simulink model "mod_win_validation"  (R2023b)
settings: Solver=FixedStepAuto  StartTime=0.0  StopTime=10  FixedStep=0.001  RelTol=1e-3
values from neighbouring files (symbols this model uses):
  atan_scale = 100    [threeDiskOscillator.m]    (also in timing_calc.m)
  b_1 = mean(ECP_values([6 7]))    [threeDiskOscillator.m]    (also in timing_calc.m)
  b_2 = mean(ECP_values([8 9]))    [threeDiskOscillator.m]    (also in timing_calc.m)
  b_3 = mean(ECP_values([10 11]))    [threeDiskOscillator.m]    (also in timing_calc.m)
  C = [  1 0 0 0 0 0 ... (first row only)    [threeDiskOscillator.m]    (also in timing_calc.m = [)
  C_kf_aug = [C zeros(3,1)]    [timing_calc.m]
  C_ref = []    [threeDiskOscillator.m]    (also in timing_calc.m = pinv(C_3*inv(eye(6) - F + G*K_discr)*G*K_discr))
  F_kf_aug = [F_d G_d(:,1);zeros(1,6) 1]    [timing_calc.m]
  G_kf_aug = [G_d;0 0]    [timing_calc.m]
  J_1 = ECP_values(1)    [threeDiskOscillator.m]    (also in timing_calc.m)
  J_2 = ECP_values(2)    [threeDiskOscillator.m]    (also in timing_calc.m)
  J_3 = ECP_values(3)    [threeDiskOscillator.m]    (also in timing_calc.m)
  k_1 = ECP_values(4)    [threeDiskOscillator.m]    (also in timing_calc.m)
  k_2 = ECP_values(5)    [threeDiskOscillator.m]    (also in timing_calc.m)
  L_kf_aug = dlqe(F_kf_aug,eye(7),C_kf_aug,1e-3*eye(7),                  sigma_meas(1,1).^2*eye(3))    [timing_calc.m]
  sigma_meas = 0.0093*eye(3)    [threeDiskOscillator.m]    (also in timing_calc.m)
  T_Cm = ECP_values(13)    [threeDiskOscillator.m]    (also in timing_calc.m)
  T_Cp = ECP_values(12)    [threeDiskOscillator.m]    (also in timing_calc.m)
  T_s = 0.004    [threeDiskOscillator.m]    (also in timing_calc.m)
  w_th = 0.75    [threeDiskOscillator.m]    (also in timing_calc.m)
  x_0 = [0;0;0;0;0;0]    [threeDiskOscillator.m]    (also in timing_calc.m)
undefined symbols (not defined in the file or in its folder): K_discr, Serial_Port, Standard_Devices
libraries: sldrtlib x3, simulink x1
settings Model: Creator=farfar  LastModifiedBy=farfar
settings DataIOCC: SaveFormat=Array  ReturnWorkspaceOutputs=off  TimeSaveName=t
settings HardwareCC: ProdBitPerLong=64  ProdHWDeviceType=Intel->x86-64 (Linux 64)
settings RTWCC: Description=Simulink Desktop Real-Time  SystemTargetFile=sldrt.tlc  TemplateMakefile=sldrt.tmf  RTWCompilerOptimization=on
settings CodeAppCC: MaxIdLength=95
settings SimulinkDesktopRealTimeCC: TargetLibSuffix=_sldrt.a  TargetPreCompLibLocation=C:\Program Files\MATLAB\R2023b\toolbox\sldrt\lib\win64

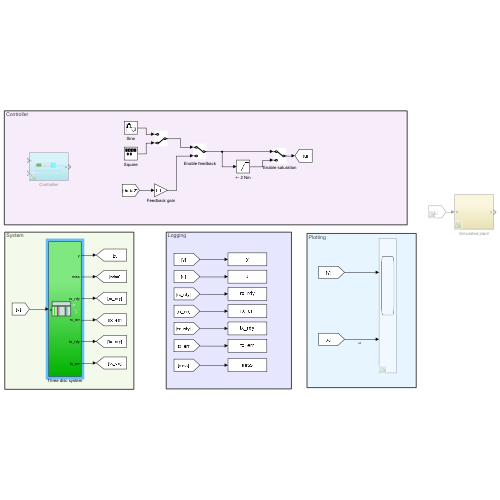
[thumbnail: Simulink's stored preview of the top-level diagram]
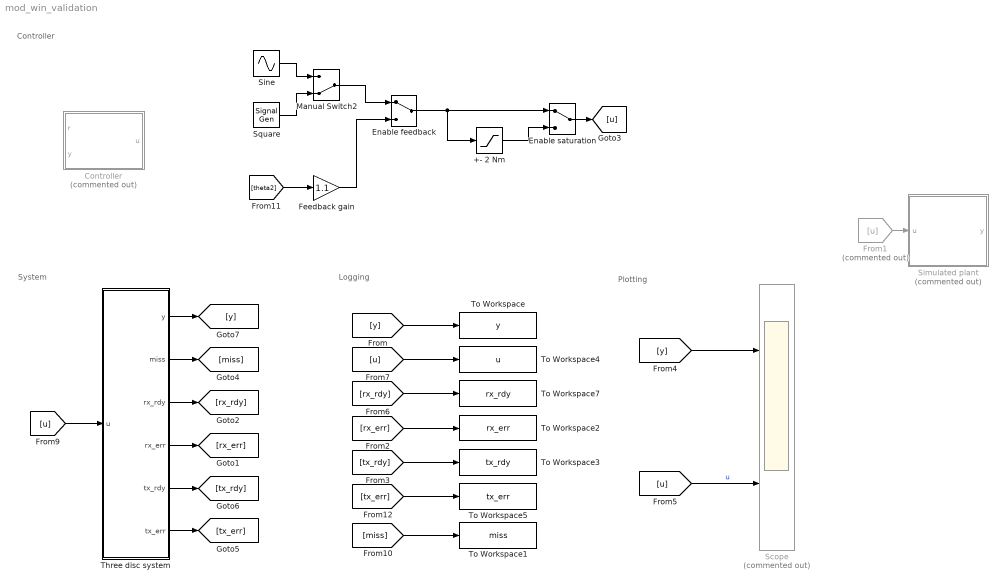
== system mod_win_validation ==
  note: Controller
  note: Plotting
  note: System
  note: Logging
  +- 2 Nm : Saturate  UpperLimit=2.0  LowerLimit=-2.0
  Controller : Subsystem  Commented=on
  Enable feedback : ManualSwitch
  Enable saturation : ManualSwitch
  Feedback gain : Gain  Gain=1.1
  From1 : From  Commented=on  GotoTag=u
  Manual Switch2 : ManualSwitch  CurrentSetting=0
  Scope : Scope  Commented=on  NumInputPorts=2
  Simulated plant : Subsystem  Commented=on
  Sine : Sin  Amplitude=0.1  Frequency=0.25*2*pi  SampleTime=0.004
  Square : SignalGenerator  WaveForm=square  Amplitude=0.1  Frequency=1/(20*0.004)
  Three disc system : Subsystem
  To Workspace : ToWorkspace  VariableName=y  SampleTime=0.001
  To Workspace1 : ToWorkspace  VariableName=miss  SampleTime=0.001
  To Workspace2 : ToWorkspace  VariableName=rx_err  SampleTime=0.001
  To Workspace3 : ToWorkspace  VariableName=tx_rdy  SampleTime=0.001
  To Workspace4 : ToWorkspace  VariableName=u  SampleTime=0.001
  To Workspace5 : ToWorkspace  VariableName=tx_err  SampleTime=0.001
  To Workspace7 : ToWorkspace  VariableName=rx_rdy  SampleTime=0.001
  wires:
  Three disc system/2(miss) -> [miss]
  Three disc system/1(y) -> [y]
  [y] -> To Workspace/1
  [u] -> To Workspace4/1
  [miss] -> To Workspace1/1
  From1/1 -> Simulated plant/1(u)
  Three disc system/3(rx_rdy) -> [rx_rdy]
  Three disc system/4(rx_err) -> [rx_err]
  [u] -> Three disc system/1(u)
  Enable feedback/1 -> Enable saturation/1, +- 2 Nm/1
  +- 2 Nm/1 -> Enable saturation/2
  Enable saturation/1 -> [u]
  [rx_rdy] -> To Workspace7/1
  Manual Switch2/1 -> Enable feedback/1
  Sine/1 -> Manual Switch2/1
  Square/1 -> Manual Switch2/2
  [theta2] -> Feedback gain/1
  Feedback gain/1 -> Enable feedback/2
  [u] -> Scope/2  "u"
  [y] -> Scope/1
  Three disc system/6(tx_err) -> [tx_err]
  Three disc system/5(tx_rdy) -> [tx_rdy]
  [rx_err] -> To Workspace2/1
  [tx_rdy] -> To Workspace3/1
  [tx_err] -> To Workspace5/1

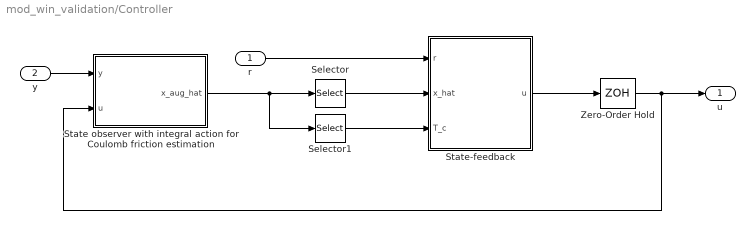
== system mod_win_validation/Controller ==
  r : Inport
  y : Inport  Port=2
  Selector : Selector  InputPortWidth=7  IndexOptions=Index vector (dialog)  Indices=[1:6]  OutputSizes=1
  Selector1 : Selector  InputPortWidth=7  IndexOptions=Index vector (dialog)  Indices=[7]  OutputSizes=1
  State observer with integral action for Coulomb friction estimation : Subsystem
  State-feedback : Subsystem
  Zero-Order Hold : ZeroOrderHold  SampleTime=T_s
  u : Outport
  wires:
  r/1 -> State-feedback/1(r)
  Zero-Order Hold/1 -> State observer with integral action for Coulomb friction estimation/2(u), u/1
  Selector1/1 -> State-feedback/3(T_c)
  Selector/1 -> State-feedback/2(x_hat)
  State-feedback/1(u) -> Zero-Order Hold/1
  y/1 -> State observer with integral action for Coulomb friction estimation/1(y)
  State observer with integral action for Coulomb friction estimation/1(x_aug_hat) -> Selector1/1, Selector/1

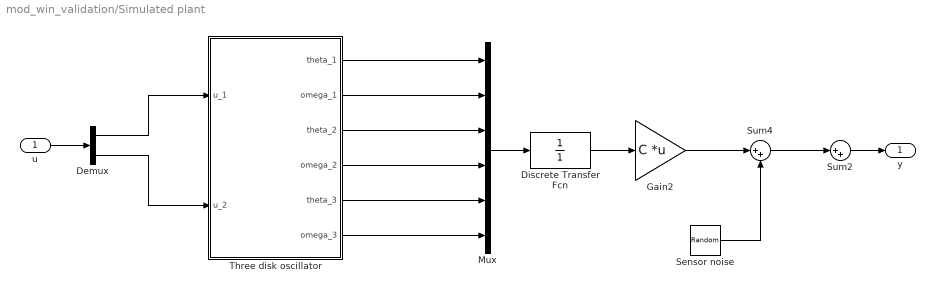
== system mod_win_validation/Simulated plant ==
  u : Inport
  Demux : Demux  Outputs=2
  Discrete Transfer Fcn : DiscreteTransferFcn  Denominator=[1]  SampleTime=T_s
  Gain2 : Gain  Gain=C  Multiplication=Matrix(K*u) (u vector)
  Mux : Mux  Inputs=6
  Sensor noise : RandomNumber  Mean=zeros(3,1)  Variance=diag(sigma_meas^2)  SampleTime=T_s
  Sum2 : Sum  Inputs=|++
  Sum4 : Sum  Inputs=|++
  Three disk oscillator : Subsystem
  y : Outport  VectorParamsAs1DForOutWhenUnconnected=off
  wires:
  u/1 -> Demux/1
  Three disk oscillator/2(omega_1) -> Mux/2
  Three disk oscillator/1(theta_1) -> Mux/1
  Mux/1 -> Discrete Transfer Fcn/1
  Three disk oscillator/4(omega_2) -> Mux/4
  Three disk oscillator/3(theta_2) -> Mux/3
  Discrete Transfer Fcn/1 -> Gain2/1
  Gain2/1 -> Sum4/1
  Sum4/1 -> Sum2/1
  Sensor noise/1 -> Sum4/2
  Three disk oscillator/6(omega_3) -> Mux/6
  Three disk oscillator/5(theta_3) -> Mux/5
  Sum2/1 -> y/1
  Demux/1 -> Three disk oscillator/1(u_1)
  Demux/2 -> Three disk oscillator/2(u_2)

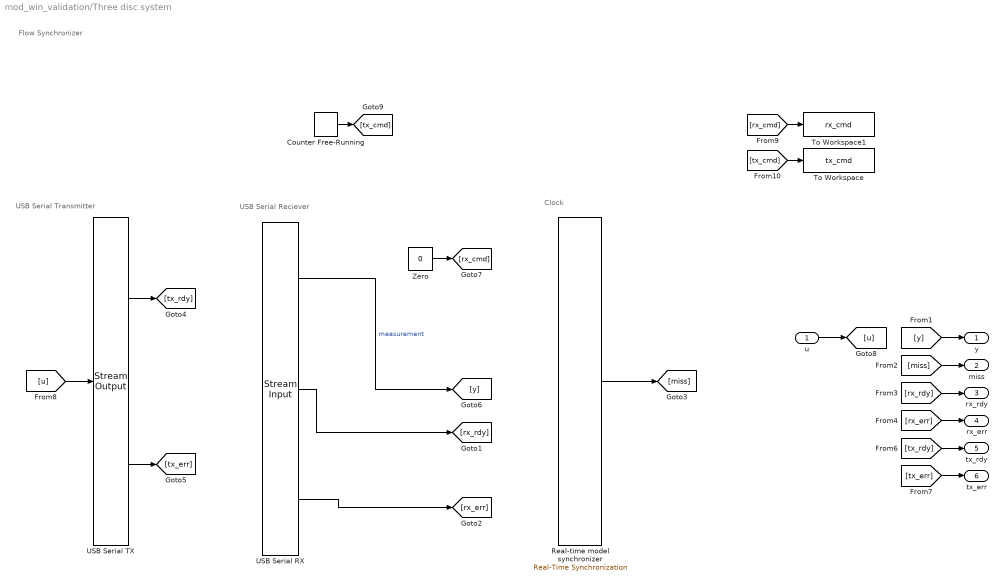
== system mod_win_validation/Three disc system ==
  note: Flow Synchronizer
  note: USB Serial Transmitter
  note: USB Serial Reciever
  note: Clock
  u : Inport
  Counter Free-Running : simulink/Sources/Counter Free-Running  NumBits=32  tsamp=0.004
  Real-time model synchronizer : sldrtlib/Real-Time Synchronization  SampleTime=0.001  MaxMissedTicks=10000  ShowMissedTicks=on  YieldWhenWaiting=off
  To Workspace : ToWorkspace  VariableName=tx_cmd  SampleTime=0.001
  To Workspace1 : ToWorkspace  VariableName=rx_cmd  SampleTime=0.001
  USB Serial RX : sldrtlib/Stream Input  SampleTime=0.001  MaxMissedTicks=10000  ShowMissedTicks=off  YieldWhenWaiting=off  DrvName=Standard_Devices/Serial_Port  DrvAddress=8  DrvOptions=[12000000 8 0 0 0 0 0 0]  DataTypes={'3*double'}  FormatString='%f %f %f'  Terminator={'\n'}  ShowReady=on  ShowError=on
      settings: AttributesFormatString=Serial Port [8]
  USB Serial TX : sldrtlib/Stream Output  SampleTime=0.004  MaxMissedTicks=1000  ShowMissedTicks=off  YieldWhenWaiting=off  DrvName=Standard_Devices/Serial_Port  DrvAddress=8  DrvOptions=[12000000 8 0 0 0 0 0 0]  PortSizes=[1]  FormatString='%f\n'  ShowReady=on  ShowError=on  InitialValue='B\n'  FinalValue='S\n'
      settings: AttributesFormatString=Serial Port [8]
  Zero : Constant  Value=0  OutDataTypeStr=Inherit: Inherit via back propagation
  y : Outport
  miss : Outport  Port=2
  rx_rdy : Outport  Port=3
  rx_err : Outport  Port=4
  tx_rdy : Outport  Port=5
  tx_err : Outport  Port=6
  wires:
  USB Serial TX/1 -> [tx_rdy]
  USB Serial RX/1 -> [y]  "measurement"
  [y] -> y/1
  u/1 -> [u]
  USB Serial RX/3 -> [rx_err]
  Real-time model synchronizer/1 -> [miss]
  [miss] -> miss/1
  [rx_rdy] -> rx_rdy/1
  [rx_err] -> rx_err/1
  USB Serial TX/2 -> [tx_err]
  [tx_err] -> tx_err/1
  [tx_rdy] -> tx_rdy/1
  [u] -> USB Serial TX/1
  Counter Free-Running/1 -> [tx_cmd]
  [rx_cmd] -> To Workspace1/1
  [tx_cmd] -> To Workspace/1
  Zero/1 -> [rx_cmd]
  USB Serial RX/2 -> [rx_rdy]

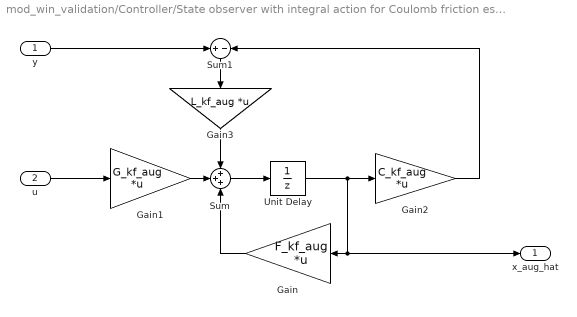
== system mod_win_validation/Controller/State observer with integral action for Coulomb friction estimation ==
  y : Inport
  u : Inport  Port=2
  Gain : Gain  Gain=F_kf_aug  Multiplication=Matrix(K*u) (u vector)
  Gain1 : Gain  Gain=G_kf_aug  Multiplication=Matrix(K*u) (u vector)
  Gain2 : Gain  Gain=C_kf_aug  Multiplication=Matrix(K*u) (u vector)
  Gain3 : Gain  Gain=L_kf_aug  Multiplication=Matrix(K*u) (u vector)
  Sum : Sum  Inputs=+++
  Sum1 : Sum  Inputs=+-
  Unit Delay : UnitDelay  SampleTime=T_s  HasFrameUpgradeWarning=on
  x_aug_hat : Outport  VectorParamsAs1DForOutWhenUnconnected=off
  wires:
  Unit Delay/1 -> x_aug_hat/1, Gain/1, Gain2/1
  y/1 -> Sum1/1
  Sum1/1 -> Gain3/1
  Sum/1 -> Unit Delay/1
  Gain2/1 -> Sum1/2
  u/1 -> Gain1/1
  Gain1/1 -> Sum/2
  Gain/1 -> Sum/3
  Gain3/1 -> Sum/1

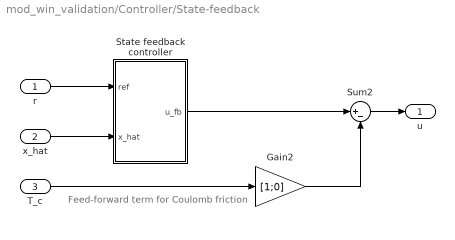
== system mod_win_validation/Controller/State-feedback ==
  note: Feed-forward term for Coulomb friction
  r : Inport
  x_hat : Inport  Port=2
  T_c : Inport  Port=3
  Gain2 : Gain  Gain=[1;0]
  State feedback controller : Subsystem
  Sum2 : Sum  Inputs=|+-
  u : Outport  VectorParamsAs1DForOutWhenUnconnected=off
  wires:
  T_c/1 -> Gain2/1
  Gain2/1 -> Sum2/2
  Sum2/1 -> u/1
  r/1 -> State feedback controller/1(ref)
  x_hat/1 -> State feedback controller/2(x_hat)
  State feedback controller/1(u_fb) -> Sum2/1

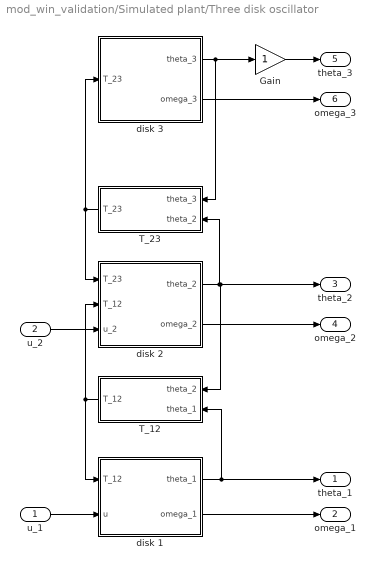
== system mod_win_validation/Simulated plant/Three disk oscillator ==
  u_1 : Inport
  u_2 : Inport  Port=2
  Gain : Gain
  T_12 : Subsystem
  T_23 : Subsystem
  disk 1 : Subsystem
  disk 2 : Subsystem
  disk 3 : Subsystem
  theta_1 : Outport  VectorParamsAs1DForOutWhenUnconnected=off
  omega_1 : Outport  Port=2  VectorParamsAs1DForOutWhenUnconnected=off
  theta_2 : Outport  Port=3  VectorParamsAs1DForOutWhenUnconnected=off
  omega_2 : Outport  Port=4  VectorParamsAs1DForOutWhenUnconnected=off
  theta_3 : Outport  Port=5  VectorParamsAs1DForOutWhenUnconnected=off
  omega_3 : Outport  Port=6  VectorParamsAs1DForOutWhenUnconnected=off
  wires:
  T_23/1(T_23) -> disk 2/1(T_23), disk 3/1(T_23)
  disk 1/1(theta_1) -> T_12/2(theta_1), theta_1/1
  disk 2/1(theta_2) -> T_23/2(theta_2), theta_2/1, T_12/1(theta_2)
  T_12/1(T_12) -> disk 1/1(T_12), disk 2/2(T_12)
  disk 3/2(omega_3) -> omega_3/1
  disk 1/2(omega_1) -> omega_1/1
  disk 2/2(omega_2) -> omega_2/1
  u_1/1 -> disk 1/2(u)
  disk 3/1(theta_3) -> Gain/1, T_23/1(theta_3)
  Gain/1 -> theta_3/1
  u_2/1 -> disk 2/3(u_2)

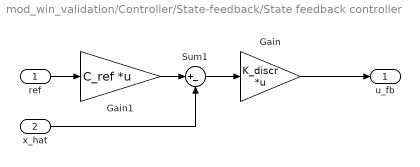
== system mod_win_validation/Controller/State-feedback/State feedback controller ==
  ref : Inport
  x_hat : Inport  Port=2
  Gain : Gain  Gain=K_discr  Multiplication=Matrix(K*u) (u vector)
  Gain1 : Gain  Gain=C_ref  Multiplication=Matrix(K*u) (u vector)
  Sum1 : Sum  Inputs=|+-
  u_fb : Outport
  wires:
  x_hat/1 -> Sum1/2
  Gain/1 -> u_fb/1
  Gain1/1 -> Sum1/1
  Sum1/1 -> Gain/1
  ref/1 -> Gain1/1

== system mod_win_validation/Simulated plant/Three disk oscillator/T_12 ==
  theta_2 : Inport
  theta_1 : Inport  Port=2
  Gain : Gain  Gain=k_1
  Sum : Sum  Inputs=|+-
  T_12 : Outport  VectorParamsAs1DForOutWhenUnconnected=off
  wires:
  theta_2/1 -> Sum/2
  theta_1/1 -> Sum/1
  Sum/1 -> Gain/1
  Gain/1 -> T_12/1

== system mod_win_validation/Simulated plant/Three disk oscillator/T_23 ==
  theta_3 : Inport
  theta_2 : Inport  Port=2
  Gain : Gain  Gain=k_2
  Sum : Sum  Inputs=-+|
  T_23 : Outport  VectorParamsAs1DForOutWhenUnconnected=off
  wires:
  Gain/1 -> T_23/1
  Sum/1 -> Gain/1
  theta_3/1 -> Sum/1
  theta_2/1 -> Sum/2

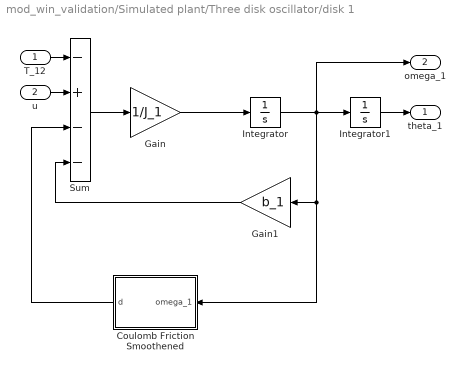
== system mod_win_validation/Simulated plant/Three disk oscillator/disk 1 ==
  T_12 : Inport
  u : Inport  Port=2
  Coulomb Friction Smoothened : Subsystem
  Gain : Gain  Gain=1/J_1
  Gain1 : Gain  Gain=b_1
  Integrator : Integrator  InitialCondition=x_0(2)
  Integrator1 : Integrator  InitialCondition=x_0(1)
  Sum : Sum  Inputs=-+--
  theta_1 : Outport  VectorParamsAs1DForOutWhenUnconnected=off
  omega_1 : Outport  Port=2  VectorParamsAs1DForOutWhenUnconnected=off
  wires:
  Sum/1 -> Gain/1
  Integrator/1 -> Integrator1/1, omega_1/1, Coulomb Friction Smoothened/1(omega_1), Gain1/1
  Gain1/1 -> Sum/4
  Integrator1/1 -> theta_1/1
  T_12/1 -> Sum/1
  u/1 -> Sum/2
  Gain/1 -> Integrator/1
  Coulomb Friction Smoothened/1(d) -> Sum/3

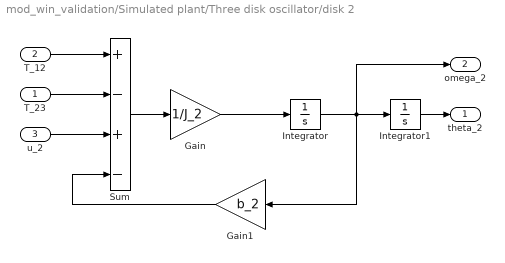
== system mod_win_validation/Simulated plant/Three disk oscillator/disk 2 ==
  T_23 : Inport
  T_12 : Inport  Port=2
  u_2 : Inport  Port=3
  Gain : Gain  Gain=1/J_2
  Gain1 : Gain  Gain=b_2
  Integrator : Integrator  InitialCondition=x_0(4)
  Integrator1 : Integrator  InitialCondition=x_0(3)
  Sum : Sum  Inputs=+-+-
  theta_2 : Outport  VectorParamsAs1DForOutWhenUnconnected=off
  omega_2 : Outport  Port=2  VectorParamsAs1DForOutWhenUnconnected=off
  wires:
  T_23/1 -> Sum/2
  T_12/1 -> Sum/1
  Integrator1/1 -> theta_2/1
  Gain1/1 -> Sum/4
  Gain/1 -> Integrator/1
  Integrator/1 -> Integrator1/1, Gain1/1, omega_2/1
  Sum/1 -> Gain/1
  u_2/1 -> Sum/3

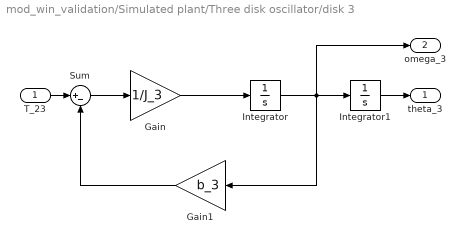
== system mod_win_validation/Simulated plant/Three disk oscillator/disk 3 ==
  T_23 : Inport
  Gain : Gain  Gain=1/J_3
  Gain1 : Gain  Gain=b_3
  Integrator : Integrator  InitialCondition=x_0(6)
  Integrator1 : Integrator  InitialCondition=x_0(5)
  Sum : Sum  Inputs=|+-
  theta_3 : Outport  VectorParamsAs1DForOutWhenUnconnected=off
  omega_3 : Outport  Port=2  VectorParamsAs1DForOutWhenUnconnected=off
  wires:
  Sum/1 -> Gain/1
  Integrator/1 -> Integrator1/1, omega_3/1, Gain1/1
  Gain/1 -> Integrator/1
  Gain1/1 -> Sum/2
  Integrator1/1 -> theta_3/1
  T_23/1 -> Sum/1

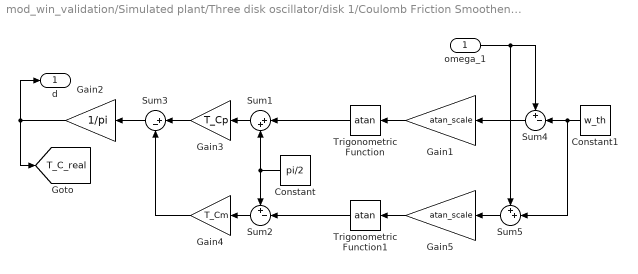
== system mod_win_validation/Simulated plant/Three disk oscillator/disk 1/Coulomb Friction Smoothened ==
  omega_1 : Inport
  Constant : Constant  Value=pi/2
  Constant1 : Constant  Value=w_th
  Gain1 : Gain  Gain=atan_scale
  Gain2 : Gain  Gain=1/pi
  Gain3 : Gain  Gain=T_Cp
  Gain4 : Gain  Gain=T_Cm
  Gain5 : Gain  Gain=atan_scale
  Sum1 : Sum  Inputs=|++
  Sum2 : Sum  Inputs=+-|
  Sum3 : Sum  Inputs=|+-
  Sum4 : Sum  Inputs=+-|
  Sum5 : Sum  Inputs=++|
  Trigonometric Function : Trigonometry  Operator=atan
  Trigonometric Function1 : Trigonometry  Operator=atan
  d : Outport  VectorParamsAs1DForOutWhenUnconnected=off
  tag scope: T_C_real=global
  wires:
  Gain1/1 -> Trigonometric Function/1
  Sum1/1 -> Gain3/1
  Constant/1 -> Sum2/1, Sum1/2
  Sum2/1 -> Gain4/1
  Sum3/1 -> Gain2/1
  Trigonometric Function/1 -> Sum1/1
  Gain4/1 -> Sum3/2
  Gain2/1 -> [T_C_real], d/1
  omega_1/1 -> Sum5/1, Sum4/1
  Gain3/1 -> Sum3/1
  Sum4/1 -> Gain1/1
  Constant1/1 -> Sum5/2, Sum4/2
  Gain5/1 -> Trigonometric Function1/1
  Sum5/1 -> Gain5/1
  Trigonometric Function1/1 -> Sum2/2
